simulink model "L2_T1_dcmotor_vs_linear"  (R2026a)
settings: Solver=ode23tb  StartTime=0  StopTime=0.3  MaxStep=0.0001
settings Model: Creator=m  LastModifiedBy=m

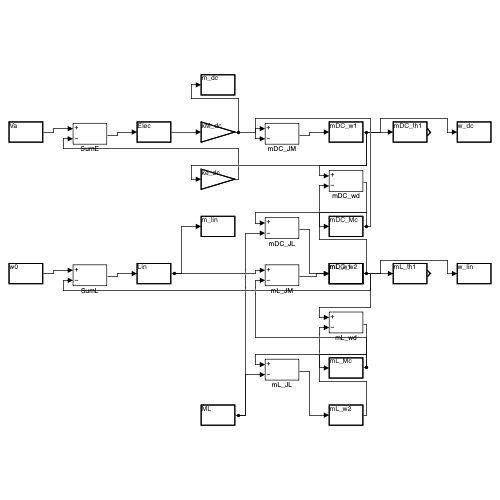
[thumbnail: Simulink's stored preview of the top-level diagram]
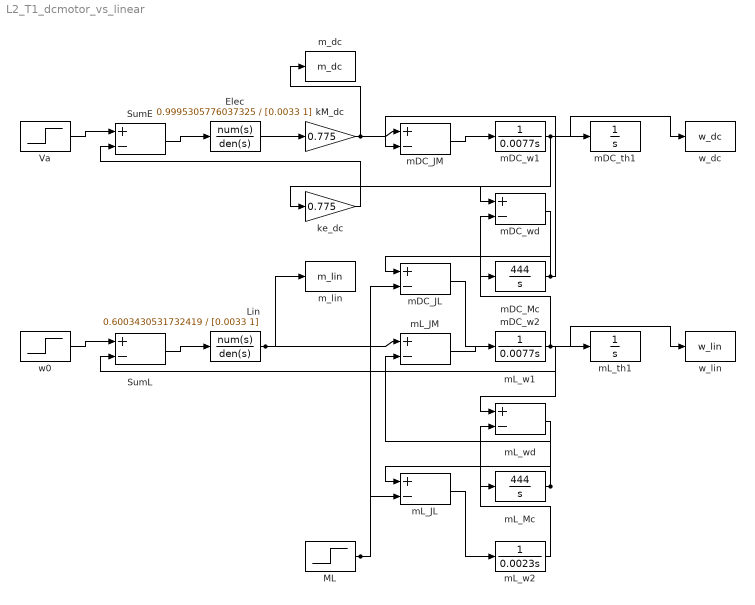
== system L2_T1_dcmotor_vs_linear ==
  Elec : TransferFcn  Numerator=0.9995305776037325  Denominator=[0.0033 1]
  Lin : TransferFcn  Numerator=0.6003430531732419  Denominator=[0.0033 1]
  ML : Step  Time=0.15  FinalValue=0.7160000000000001  SampleTime=0
  SumE : Sum  Inputs=+-
  SumL : Sum  Inputs=+-
  Va : Step  Time=0  FinalValue=90.36499999999999  SampleTime=0
  kM_dc : Gain  Gain=0.775
  ke_dc : Gain  Gain=0.775
  mDC_JL : Sum  Inputs=+-
  mDC_JM : Sum  Inputs=+-
  mDC_Mc : TransferFcn  Numerator=444  Denominator=[1 0]
  mDC_th1 : Integrator
  mDC_w1 : TransferFcn  Numerator=1  Denominator=[0.0077 0]
  mDC_w2 : TransferFcn  Numerator=1  Denominator=[0.0023 0]
  mDC_wd : Sum  Inputs=+-
  mL_JL : Sum  Inputs=+-
  mL_JM : Sum  Inputs=+-
  mL_Mc : TransferFcn  Numerator=444  Denominator=[1 0]
  mL_th1 : Integrator
  mL_w1 : TransferFcn  Numerator=1  Denominator=[0.0077 0]
  mL_w2 : TransferFcn  Numerator=1  Denominator=[0.0023 0]
  mL_wd : Sum  Inputs=+-
  m_dc : ToWorkspace  VariableName=m_dc  SaveFormat=Structure With Time  SampleTime=-1
  m_lin : ToWorkspace  VariableName=m_lin  SaveFormat=Structure With Time  SampleTime=-1
  w0 : Step  Time=0  FinalValue=116.6  SampleTime=0
  w_dc : ToWorkspace  VariableName=w_dc  SaveFormat=Structure With Time  SampleTime=-1
  w_lin : ToWorkspace  VariableName=w_lin  SaveFormat=Structure With Time  SampleTime=-1
  wires:
  mDC_JM/1 -> mDC_w1/1
  mDC_w1/1 -> mDC_wd/1, mDC_th1/1, ke_dc/1, w_dc/1
  mDC_w2/1 -> mDC_wd/2
  mDC_wd/1 -> mDC_Mc/1
  mDC_Mc/1 -> mDC_JM/2, mDC_JL/1
  mDC_JL/1 -> mDC_w2/1
  Va/1 -> SumE/1
  ke_dc/1 -> SumE/2
  SumE/1 -> Elec/1
  Elec/1 -> kM_dc/1
  kM_dc/1 -> mDC_JM/1, m_dc/1
  ML/1 -> mDC_JL/2, mL_JL/2
  mL_JM/1 -> mL_w1/1
  mL_w1/1 -> mL_wd/1, mL_th1/1, SumL/2, w_lin/1
  mL_w2/1 -> mL_wd/2
  mL_wd/1 -> mL_Mc/1
  mL_Mc/1 -> mL_JM/2, mL_JL/1
  mL_JL/1 -> mL_w2/1
  w0/1 -> SumL/1
  SumL/1 -> Lin/1
  Lin/1 -> mL_JM/1, m_lin/1
